simulink model "Q2sim4"  (R2022a)
settings: Solver=VariableStepAuto  StartTime=0.0  StopTime=30  FixedStep=1e-4  RelTol=1e-3
values from neighbouring files (symbols this model uses):
  A = [0 1  0              0 ... (first row only)    [Q2.m]
  Am = M    (= 0)    [Q2.m]
  B = [0; 1/M; 0; -1/(M*L)]    [Q2.m]
  Bm = N    (= 1)    [Q2.m]
  C = [1 0 0 0]    [Q2.m]
  Dsim = zeros(4,1)    [Q2.m]
  K = Ka (1:4)    [Q2.m]
  Km = Ka(5)    [Q2.m]
  L = lqr(A',C',Ql,Rl)'    [Q2.m]
  x0 = [0 0 deg2rad(51) 0]    [Q2.m]
  x0obs = [0 0 0 0]    [Q2.m]
settings Model: Creator=Crippa  LastModifiedBy=Crippa
settings SolverCC: ZeroCrossControl=DisableAll

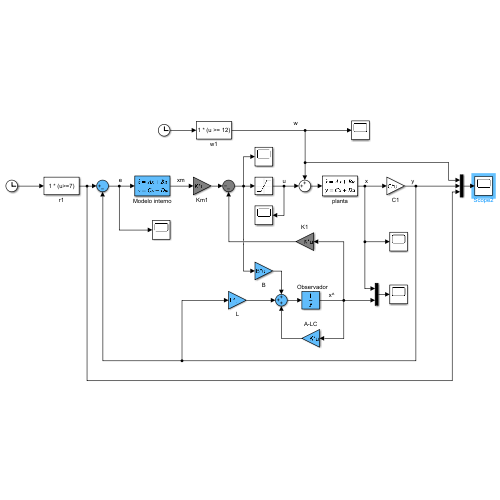
[thumbnail: Simulink's stored preview of the top-level diagram]
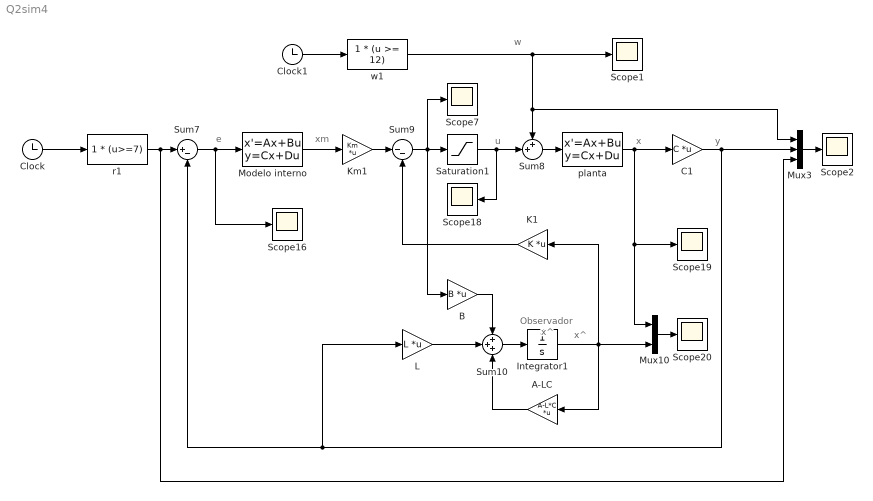
== system Q2sim4 ==
  note: w
  note: u
  note: x
  note: xm
  note: Observador
  note: x^
  note: e
  note: y
  note: x^
  A-LC : Gain  Gain=A-L*C  Multiplication=Matrix(K*u)
  B : Gain  Gain=B  Multiplication=Matrix(K*u)
  C1 : Gain  Gain=C  Multiplication=Matrix(K*u)
  Clock : Clock
  Clock1 : Clock
  Integrator1 : Integrator  InitialCondition=x0obs
  K1 : Gain  Gain=K  Multiplication=Matrix(K*u)
  Km1 : Gain  Gain=Km  Multiplication=Matrix(K*u)
  L : Gain  Gain=L  Multiplication=Matrix(K*u)
  Modelo interno : StateSpace  A=Am  B=Bm  C=eye(1)  D=zeros(1)  InitialCondition=0
  Mux10 : Mux  Inputs=2
  Mux3 : Mux  Inputs=3
  Saturation1 : Saturate  UpperLimit=150  LowerLimit=-150
  Scope{1..2,7,16,18..20} (7 alike) : Scope
  Sum10 : Sum  Inputs=+++
  Sum7 : Sum  Inputs=|+-
  Sum8 : Sum  Inputs=++|
  Sum9 : Sum  Inputs=|--
  planta : StateSpace  A=A  B=B  C=eye(4)  D=Dsim  InitialCondition=x0
  r1 : Fcn  Expr=1 * (u>=7)
  w1 : Fcn  Expr=1 * (u >= 12)
  wires:
  Mux3/1 -> Scope2/1
  Clock1/1 -> w1/1
  w1/1 -> Scope1/1, Mux3/1, Sum8/1
  Sum10/1 -> Integrator1/1
  Mux10/1 -> Scope20/1
  K1/1 -> Sum9/2
  Integrator1/1 -> Mux10/2, A-LC/1, K1/1
  C1/1 -> Mux3/2, L/1, Sum7/2
  B/1 -> Sum10/1
  A-LC/1 -> Sum10/3
  Sum7/1 -> Modelo interno/1, Scope16/1
  Km1/1 -> Sum9/1
  Saturation1/1 -> Sum8/2, Scope18/1
  r1/1 -> Mux3/3, Sum7/1
  Sum9/1 -> Scope7/1, B/1, Saturation1/1
  L/1 -> Sum10/2
  Modelo interno/1 -> Km1/1
  planta/1 -> C1/1, Scope19/1, Mux10/1
  Sum8/1 -> planta/1
  Clock/1 -> r1/1
